simulink model "B1P6_Torsonal_Model_2_Coupler"  (Simulink 6.4)
settings: Solver=ode23tb  StartTime=0.0  StopTime=0.5  RelTol=1e-3
values from neighbouring files (symbols this model uses):
  B1 = 0    [B1P3_Torsonal_Model_1_Coupler_Constants.m]    (also in B1P6_Torsonal_Model_2_Coupler_Constants.m; Torsonal_Model_Constants.m)
  B2 = 0    [B1P6_Torsonal_Model_2_Coupler_Constants.m]
  B3 = 0    [B1P6_Torsonal_Model_2_Coupler_Constants.m]
  Bc1 = 0.01    [B1P6_Torsonal_Model_2_Coupler_Constants.m]
  Bc2 = 0.01    [B1P6_Torsonal_Model_2_Coupler_Constants.m]
  J1 = 0.0033    [B1P3_Torsonal_Model_1_Coupler_Constants.m]    (also in B1P6_Torsonal_Model_2_Coupler_Constants.m = 0.0023; Torsonal_Model_Constants.m = 0.0023)
  J2 = J1/2    (= 0.00115)    [B1P6_Torsonal_Model_2_Coupler_Constants.m]
  J3 = .0023E0    (= 0.0023)    [B1P6_Torsonal_Model_2_Coupler_Constants.m]
  Kc1 = 100000    [B1P6_Torsonal_Model_2_Coupler_Constants.m]
  Kc2 = 1000    [B1P6_Torsonal_Model_2_Coupler_Constants.m]
settings Model: Creator=dml46  LastModifiedBy=Geovana
settings DebuggingCC: MultiTaskDSMMsg=error  MultiTaskCondExecSysMsg=error

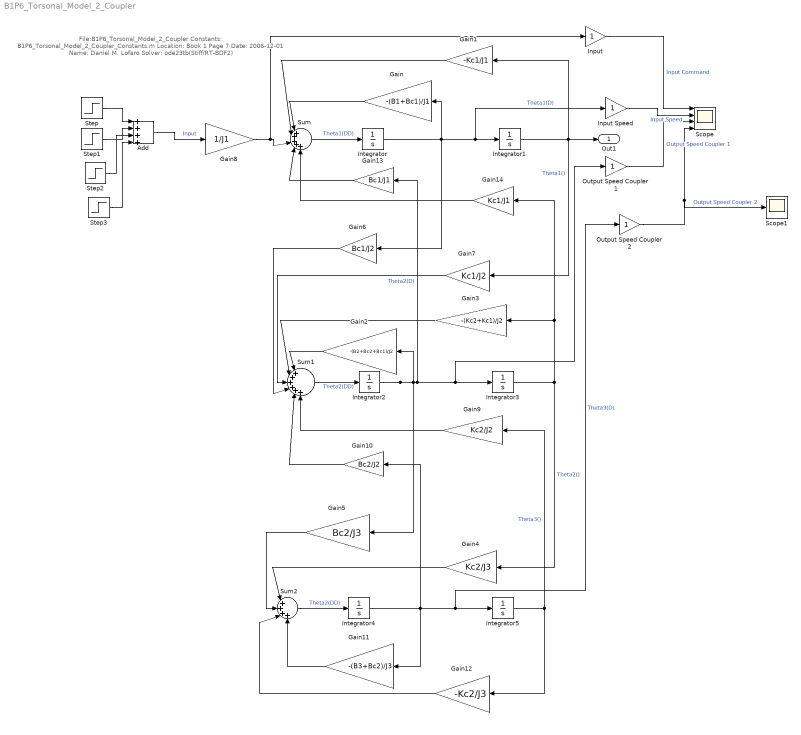
== system B1P6_Torsonal_Model_2_Coupler ==
  note: File:B1P6_Torsonal_Model_2_Coupler
      | Constants: B1P6_Torsonal_Model_2_Coupler_Constants.m
      | Location: Book 1 Page 7
      | Date: 2006-12-01
      | Name: Daniel M. Lofaro
      | Solver: ode23tb(Stiff/RT-BDF2)
  Add : Sum  Inputs=++++  OutScaling=2^-10
  Gain : Gain  Orientation=left  Gain=-(B1+Bc1)/J1
  Gain1 : Gain  Orientation=left  Gain=-Kc1/J1
  Gain10 : Gain  Orientation=left  Gain=Bc2/J2
  Gain11 : Gain  Orientation=left  Gain=-(B3+Bc2)/J3
  Gain12 : Gain  Orientation=left  Gain=-Kc2/J3
  Gain13 : Gain  Orientation=left  Gain=Bc1/J1
  Gain14 : Gain  Orientation=left  Gain=Kc1/J1
  Gain2 : Gain  Orientation=left  Gain=-(B2+Bc2+Bc1)/J2
  Gain3 : Gain  Orientation=left  Gain=-(Kc2+Kc1)/J2
  Gain4 : Gain  Orientation=left  Gain=Kc2/J3
  Gain5 : Gain  Orientation=left  Gain=Bc2/J3
  Gain6 : Gain  Orientation=left  Gain=Bc1/J2
  Gain7 : Gain  Orientation=left  Gain=Kc1/J2
  Gain8 : Gain  Gain=1/J1
  Gain9 : Gain  Orientation=left  Gain=Kc2/J2
  Input : Gain
  Input Speed : Gain
  Integrator{,1..5} (6 alike) : Integrator
  Output Speed Coupler 1 : Gain
  Output Speed Coupler 2 : Gain
  Scope : Scope  NumInputPorts=4
      settings: YMin=-5~-5~-5~-5  YMax=5~5~5~5
  Scope1 : Scope
  Step : Step  Time=0.1  SampleTime=0
  Step1 : Step  Time=0.2  After=-1  SampleTime=0
  Step2 : Step  Time=0.3  After=-1  SampleTime=0
  Step3 : Step  Time=0.4  SampleTime=0
  Sum : Sum  Inputs=|+++++
  Sum1 : Sum  Inputs=|++++++
  Sum2 : Sum  Inputs=|++++
  Out1 : Outport
  wires:
  Step/1 -> Add/1
  Step1/1 -> Add/2
  Step2/1 -> Add/3
  Step3/1 -> Add/4
  Sum2/1 -> Integrator4/1  "Theta2(DD)"
  Sum1/1 -> Integrator2/1  "Theta2(DD)"
  Sum/1 -> Integrator/1  "Theta1(DD)"
  Integrator/1 -> Gain/1, Gain6/1, Integrator1/1, Input Speed/1  "Theta1(D)"
  Integrator2/1 -> Gain13/1, Integrator3/1, Output Speed Coupler 1/1, Gain2/1, Gain5/1  "Theta2(D)"
  Integrator4/1 -> Gain10/1, Gain11/1, Integrator5/1, Output Speed Coupler 2/1  "Theta3(D)"
  Gain8/1 -> Sum/3, Input/1
  Gain/1 -> Sum/1
  Gain1/1 -> Sum/2
  Integrator1/1 -> Gain1/1, Gain7/1, Out1/1  "Theta1()"
  Gain14/1 -> Sum/5
  Integrator3/1 -> Gain14/1, Gain3/1, Gain4/1  "Theta2()"
  Gain13/1 -> Sum/4
  Gain6/1 -> Sum1/4
  Gain7/1 -> Sum1/3
  Gain2/1 -> Sum1/1
  Gain3/1 -> Sum1/2
  Gain9/1 -> Sum1/6
  Gain10/1 -> Sum1/5
  Integrator5/1 -> Gain9/1, Gain12/1  "Theta3()"
  Gain4/1 -> Sum2/1
  Gain5/1 -> Sum2/2
  Gain11/1 -> Sum2/4
  Gain12/1 -> Sum2/3
  Input/1 -> Scope/1  "Input Command"
  Input Speed/1 -> Scope/2  "Input Speed"
  Output Speed Coupler 1/1 -> Scope/3  "Output Speed Coupler 1"
  Output Speed Coupler 2/1 -> Scope/4, Scope1/1  "Output Speed Coupler 2"
  Add/1 -> Gain8/1  "Input"
